simulink model "mass_spring_damper"  (R2024b)
settings: Solver=VariableStepAuto  StartTime=0.0  StopTime=30  MaxStep=0.01  RelTol=1e-3
settings Model: Creator=Aryan  LastModifiedBy=Aryan

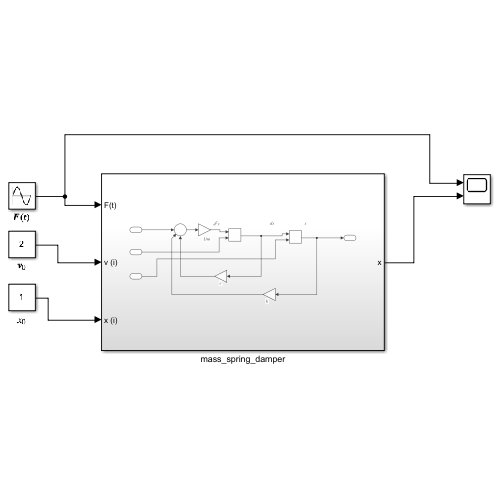
[thumbnail: Simulink's stored preview of the top-level diagram]
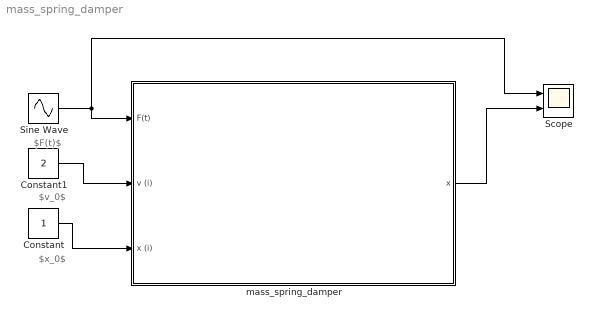
== system mass_spring_damper ==
  note: $F(t)$
  note: $x_0$
  note: $v_0$
  Constant : Constant
  Constant1 : Constant  Value=2
  Scope : Scope  NumInputPorts=2
  Sine Wave : Sin  Amplitude=2  Frequency=2  SampleTime=0
  mass_spring_damper : Subsystem
  wires:
  Sine Wave/1 -> Scope/1, mass_spring_damper/1(F(t))
  Constant1/1 -> mass_spring_damper/2(v (i))
  Constant/1 -> mass_spring_damper/3(x (i))
  mass_spring_damper/1(x) -> Scope/2

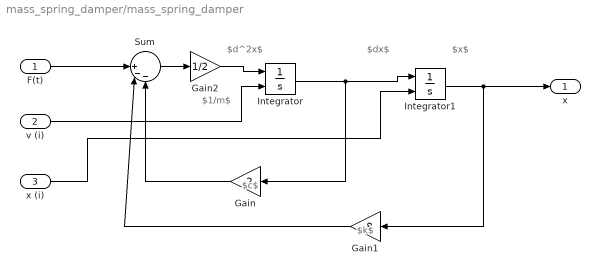
== system mass_spring_damper/mass_spring_damper ==
  note: $1/m$
  note: $k$
  note: $c$
  note: $x$
  note: $dx$
  note: $d^2x$
  F(t) : Inport
  v (i) : Inport  Port=2
  x (i) : Inport  Port=3
  Gain : Gain  Gain=2
  Gain1 : Gain  Gain=8
  Gain2 : Gain  Gain=1/2
  Integrator : Integrator  InitialConditionSource=external  InitialCondition=2
  Integrator1 : Integrator  InitialConditionSource=external  InitialCondition=1
  Sum : Sum  Inputs=||+--
  x : Outport
  wires:
  F(t)/1 -> Sum/1
  Integrator1/1 -> x/1, Gain1/1
  Gain/1 -> Sum/3
  Gain2/1 -> Integrator/1
  Integrator/1 -> Integrator1/1, Gain/1
  Gain1/1 -> Sum/2
  Sum/1 -> Gain2/1
  x (i)/1 -> Integrator1/2
  v (i)/1 -> Integrator/2
